simulink model "ex3"  (R2021b)
settings: Solver=VariableStepAuto  StartTime=0.0  StopTime=10.0  RelTol=1e-3

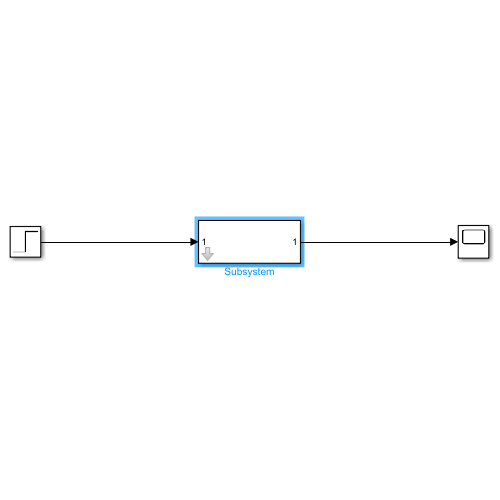
[thumbnail: Simulink's stored preview of the top-level diagram]
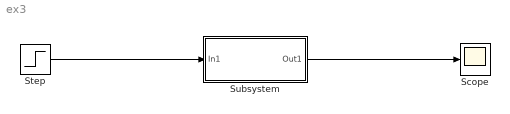
== system ex3 ==
  Scope : Scope
  Step : Step  SampleTime=0
  Subsystem : Subsystem  mask{a=3}
      mask init:
      | a = str2num(get_param(gcb, 'a'));
      | if a < 2 || a > 4
      |     error('valoarea parametrului a trebuie sa fie in intervalul [2;4]')
      | end
  wires:
  Step/1 -> Subsystem/1(In1)
  Subsystem/1(Out1) -> Scope/1

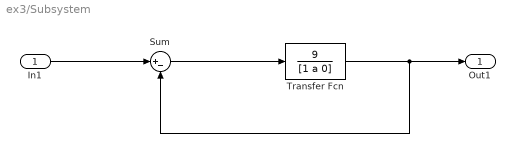
== system ex3/Subsystem ==
  In1 : Inport
  Sum : Sum  Inputs=|+-
  Transfer Fcn : TransferFcn  Numerator=[9]  Denominator=[1 a 0]
  Out1 : Outport
  wires:
  In1/1 -> Sum/1
  Sum/1 -> Transfer Fcn/1
  Transfer Fcn/1 -> Sum/2, Out1/1
